simulink model "Statechart_Test_2"  (R2016b)
settings: Solver=ode45  StartTime=0.0  StopTime=100  RelTol=1e-3  EnableMultiTasking=on
PreLoadFcn:
  | RED = 0;
  | ORANGE = 1;
  | GREEN = 2;
settings Model: Creator=The MathWorks, Inc.  LastModifiedBy=Rose
settings DataIOCC: LimitDataPoints=on  SaveFormat=Array
settings OptimizationCC: ExpressionDepthLimit=2147483647  LifeSpan=1
settings DebuggingCC: UnderspecifiedInitializationDetection=Classic  MergeDetectMultiDrivingBlocksExec=none  FcnCallInpInsideContextMsg=warning  StateNameClashWarn=warning  SFUnexpectedBacktrackingDiag=warning  SFNoUnconditionalDefaultTransitionDiag=warning  SFExecutionAtInitializationDiag=none
settings HardwareCC: ProdBitPerPointer=32  ProdBitPerSizeT=32  ProdBitPerPtrDiffT=32  ProdLargestAtomicFloat=None  ProdIntDivRoundTo=Undefined  ProdEndianess=Unspecified  ProdWordSize=32  ProdHWDeviceType=32-bit Generic
settings ModelReferenceCC: PropagateSignalLabelsOutOfModel=off
settings RTWCC: SystemTargetFile=ert.tlc  TemplateMakefile=ert_default_tmf  Description=Embedded Coder
settings CodeAppCC: IgnoreCustomStorageClasses=off  CustomSymbolStrType=$N$R$M  InternalIdentifier=Classic
settings ERTTargetCC: GenerateSampleERTMain=on  ERTCustomFileTemplate=example_file_process.tlc  ConvertIfToSwitch=off  SuppressUnreachableDefaultCases=off
settings ConfigComp: CovMetricSettings=dw  CovHtmlReporting=on  CovSaveCumulativeToWorkspaceVar=on  CovSaveSingleToWorkspaceVar=on  CovExternalEMLEnable=off

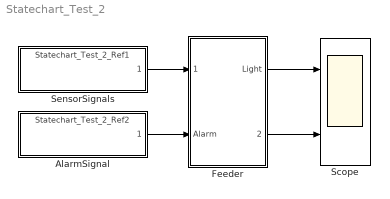
== system Statechart_Test_2 ==
  AlarmSignal : ModelReference  ModelNameDialog=Statechart_Test_2_Ref2  SimulationMode=Normal  ModelReferenceVersion=1.48
  Feeder : Stateflow chart  TreatAsAtomicUnit=on
  Scope : Scope  NumInputPorts=2
  SensorSignals : ModelReference  ModelNameDialog=Statechart_Test_2_Ref1  SimulationMode=Normal  ModelReferenceVersion=1.48
  wires:
  SensorSignals/1 -> Feeder/1(sensors)
  Feeder/1(Light) -> Scope/1
  AlarmSignal/1 -> Feeder/2(Alarm)
  Feeder/2(partsFed) -> Scope/2

== stateflow chart Statechart_Test_2/Feeder ==
  state InitializeSystem
    entry:
    Light = ORANGE;
  state FailState
    entry:
    Light = RED;
  state On
    entry:
    Light = GREEN;
    partsFed = 0;
    during:
    if(any(sensors >= 2))
    partsFed = partsFed + 1;
    end
  (default) -> InitializeSystem
  FailState -> InitializeSystem : [Alarm == 0]
  InitializeSystem -> FailState [order 2] : after(5,sec)
  InitializeSystem -> On [order 1] : [all(sensors>0)]
  On -> FailState : [Alarm ==1]
  data: sensors input; Alarm input; Light output; partsFed output; GREEN parameter; ORANGE parameter; RED parameter
